simulink model "PID1_example"  (R2015b)
settings: Solver=VariableStepAuto  StartTime=0.0  StopTime=10.0  RelTol=1e-3
settings Model: Creator=mctra  LastModifiedBy=mctra

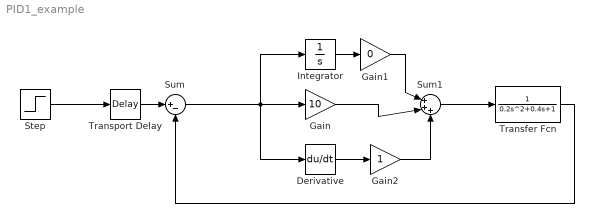
== system PID1_example ==
  Derivative : Derivative
  Gain : Gain  Gain=10
  Gain1 : Gain  Gain=0
  Gain2 : Gain
  Integrator : Integrator
  Step : Step  SampleTime=0
  Sum : Sum  Inputs=|+-
  Sum1 : Sum  Inputs=|+++
  Transfer Fcn : TransferFcn  Numerator=1  Denominator=[0.2 0.4 1]
  Transport Delay : TransportDelay  DelayTime=0.209
  wires:
  Sum1/1 -> Transfer Fcn/1
  Transport Delay/1 -> Sum/1
  Transfer Fcn/1 -> Sum/2
  Step/1 -> Transport Delay/1
  Integrator/1 -> Gain1/1
  Derivative/1 -> Gain2/1
  Sum/1 -> Derivative/1, Integrator/1, Gain/1
  Gain1/1 -> Sum1/1
  Gain/1 -> Sum1/2
  Gain2/1 -> Sum1/3
